simulink model "Non_Linear_plant"  (R2024b)
settings: Solver=VariableStepAuto  StartTime=0.0  StopTime=300  RelTol=1e-3
settings Model: Creator=aryaman  LastModifiedBy=aryaman
settings DataIOCC: SaveFormat=StructureWithTime

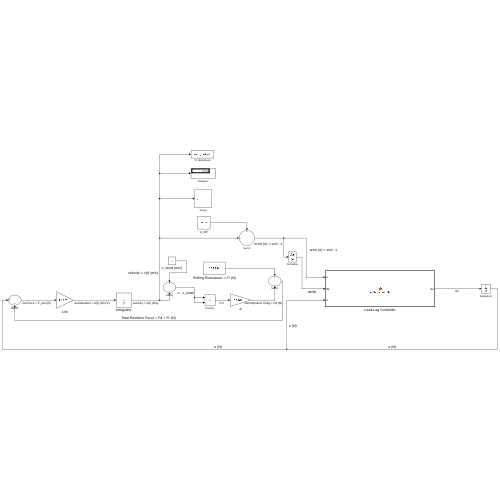
[thumbnail: Simulink's stored preview of the top-level diagram]
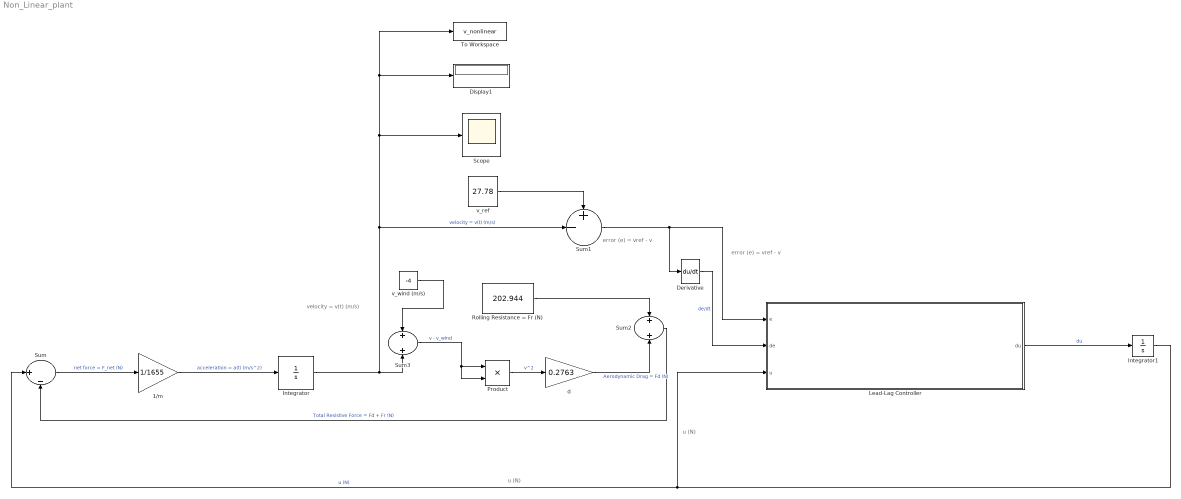
== system Non_Linear_plant ==
  note: u (N)
  note: u (N)
  note: velocity = v(t) (m/s)
  note: error (e) = vref - v
  note: error (e) = vref - v
  1/m : Gain  Gain=1/1655
  Derivative : Derivative
  Display1 : Display
  Integrator : Integrator
  Integrator1 : Integrator
  Lead-Lag Controller : MATLAB Function  TreatAsAtomicUnit=on
  Product : Product
  Rolling Resistance = Fr (N) : Constant  Value=202.944
  Scope : Scope
  Sum : Sum  Inputs=||+|-
  Sum1 : Sum  Inputs=+-|
  Sum2 : Sum  Inputs=+|+
  Sum3 : Sum  Inputs=+|+
  To Workspace : ToWorkspace  VariableName=v_nonlinear  SampleTime=-1
  d : Gain  Gain=0.2763
  v_ref : Constant  Value=27.78
  v_wind (m/s) : Constant  Value=-4
  wires:
  Sum/1 -> 1/m/1  "net force = F_net (N)"
  1/m/1 -> Integrator/1  "acceleration = a(t) (m/s^2)"
  Integrator/1 -> Sum3/2, Sum1/2, Scope/1, To Workspace/1, Display1/1  "velocity = v(t) (m/s)"
  v_ref/1 -> Sum1/1
  Sum1/1 -> Derivative/1, Lead-Lag Controller/1(e)
  Derivative/1 -> Lead-Lag Controller/2(de)  "de/dt"
  Lead-Lag Controller/1(du) -> Integrator1/1  "du"
  Integrator1/1 -> Lead-Lag Controller/3(u), Sum/1  "u (N)"
  Product/1 -> d/1  "v^2"
  Rolling Resistance = Fr (N)/1 -> Sum2/1
  d/1 -> Sum2/2  "Aerodynamic Drag = Fd (N)"
  Sum2/1 -> Sum/2  "Total Resistive Force = Fd + Fr (N)"
  v_wind (m/s)/1 -> Sum3/1
  Sum3/1 -> Product/2, Product/1  "v - v_wind"

== matlab function Non_Linear_plant/Lead-Lag Controller ==
  data: e input; du output; de input; u input
function du = leadlag_controller(e, de, u)
% e = error = v_ref - v

% Controller parameters
%K = 100;
%z = 2.50;
%p = 0.020;

K = 50;
z = 2.40;
p = 0.050;

% Lead-Lag Transfer Function
% C(s) = U(s)/E(s)
%C = K * (s + z) / (s + p);

du = K*(de + z*e) - p*u;

end
